simulink model "testemplanner_cs"  (R2020a)
settings: Solver=ode5  StartTime=0.0  StopTime=30  FixedStep=1/1000  RelTol=1e-3
PreLoadFcn:
  | mbxruntime.callbacks.PreLoadFcn(bdroot);
PostLoadFcn:
  | mbxruntime.callbacks.PostLoadFcn(bdroot);
InitFcn:
  | mbxruntime.callbacks.InitFcn(bdroot);
StartFcn:
  | mbxruntime.callbacks.StartFcn(bdroot);
StopFcn:
  | mbxruntime.callbacks.StopFcn(bdroot);
model workspace (MAT data in the model file):
  mbox_table : object (value not decoded)
  model_closed = 0
  sim_status = 0
values from neighbouring files (symbols this model uses):
  c_factor = 43.75    [emplanner_init.m]
  cf = -175016    [emplanner_init.m]
  cr = -130634    [emplanner_init.m]
  global_path_x = [-12.787 -11.7876177449 -10.7894946344 -9.79264775065 -8.79708287721 -7.80280164192 -6.80980414431 -5.81808992236 -4.82765830817 -3.83850855887 -2.85063990477 -1.86405156707 ... (3001 elements, 3001x1)]    [global_path.mat]
  global_path_y = [5.7602 5.7602 5.7602 5.7602 5.7602 5.7602 5.7602 5.7602 5.7602 5.7602 5.7602 5.7602 ... (3001 elements, 3001x1)]    [global_path.mat]
  KD_PID_distance = 0.0    (= 0)    [emplanner_init.m]
  KD_PID_speed = 0    [emplanner_init.m]
  KI_PID_distance = 0.0    (= 0)    [emplanner_init.m]
  KI_PID_speed = 0    [emplanner_init.m]
  KP_PID_distance = 0.5    [emplanner_init.m]
  KP_PID_speed = 1.8    [emplanner_init.m]
  la = 1.265    [emplanner_init.m]
  lb = 2.947-1.265    (= 1.682)    [emplanner_init.m]
  LQR_K1 = k(:,1)'    [emplanner_init.m]
  LQR_K2 = k(:,2)'    [emplanner_init.m]
  LQR_K3 = k(:,3)'    [emplanner_init.m]
  LQR_K4 = k(:,4)'    [emplanner_init.m]
  m = 2020    [emplanner_init.m]
  rack_displacement = [-39.14 , -37.2 , -35.29 , -33.43 , -31.6 , -29.81 , -28.06 , -26.34 , -24.66 ,      -23.01 , -21.38 , -19.79 , -18.23 , -16.69 , -15.18 , -13.7 , -12.23 , -10.8 , -9.38 , -7.98 ,     -6.61 , -5.25 , -3.91 , -2.59 , -1.29 , 0 , 1.27 , 2.54 , 3.78 , 5.02 , 6.24 , 7.46 , 8.66 ,      9.86 , 11.05 , 12.24 , 13.41 , 14.59 , 15.76 , 16.92 , 18.09 , 19.25 , 20.42 , 21.59 , 22.76 ,      23.93 , 25.11 , 26 ...(+26 chars)    [emplanner_init.m]
  right_wheel_ground = [-70 ,-67.2 , -64.4 , -61.6 , -58.8 , -56 , -53.2 , -50.4 , -47.6 , -44.8 , -42 ,      -39.2 , -36.4 , -33.6 , -30.8 , -28 , -25.2 , -22.4 , -19.6 , -16.8 , -14 , -11.2 , -8.4 , -5.6 ,      -2.8 , 0 , 2.8 , 5.6 , 8.4 , 11.2 , 14 , 16.8 , 19.6 , 22.4 , 25.2 , 28 , 30.8 , 33.6 , 36.4 ,      39.2 , 42 , 44.8 , 47.6 , 50.4 , 53.2 , 56 , 58.8 , 61.6 , 64.4 , 67.2 , 70 ]    [emplanner_init.m]
  vx_break_point = zeros(1,5000)    [emplanner_init.m]
undefined symbols (not defined in the file or in its folder): aubr, DiscIntNeverNeededParam, tablebr, vubr, warningInitialVelocity, x0
libraries: PreScanSimulinkLibrary x39, simulink x19, simulink_extras x11, Solver_SF x1
(part 5 of 16)

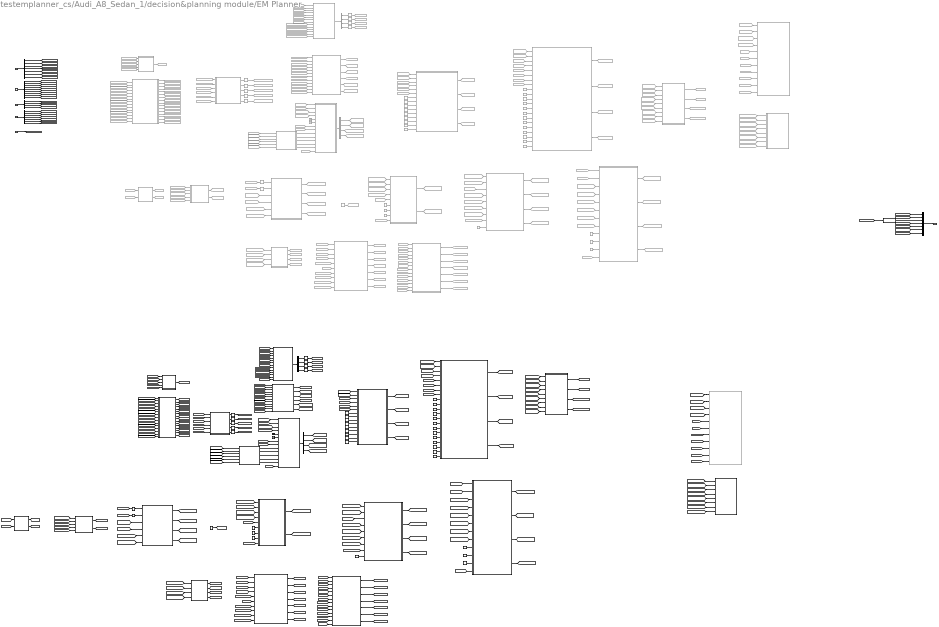
== system testemplanner_cs/Audi_A8_Sedan_1/decision&planning module/EM Planner ==
  referenceline info : Inport
  location info : Inport  Port=2
  perception info : Inport  Port=3
  pre_planning info : Inport  Port=4
  current time : Inport  Port=5
  Bus Creator : BusCreator  Inputs=7
  Bus Selector : BusSelector  OutputSignals=referenceline_x,referenceline_y,referenceline_heading,referenceline_kappa,origin_match_point_index,origin_x,origin_y
  Bus Selector1 : BusSelector  OutputSignals=host_x,host_y,host_heading_xy,host_vx,host_vy,host_yawrate,host_speed,host_ax,host_ay
  Bus Selector2 : BusSelector  OutputSignals=obs_x_set_gcs,obs_y_set_gcs,obs_velocity_set_gcs,obs_heading_set_gcs
  Bus Selector3 : BusSelector  OutputSignals=trajectory_x_gcs,trajectory_y_gcs,trajectory_heading_gcs,trajectory_kappa_gcs,trajectory_speed_gcs,trajectory_accel_gcs,trajectory_time_gcs
  Bus Selector4 : BusSelector  Commented=on  OutputSignals=s_set,l_set,dl_set,ddl_set
  Bus Selector5 : BusSelector  Commented=on  OutputSignals=s_set,l_set,s_dot_set,l_dot_set
  Bus Selector6 : BusSelector  OutputSignals=s_set,l_set,dl_set,ddl_set
  Bus Selector7 : BusSelector  OutputSignals=s_set,l_set,s_dot_set,l_dot_set
  Cartesian2Frenet : Subsystem  Commented=on
  Cartesian2Frenet1 : Subsystem  Commented=on
  Cartesian2Frenet2 : Subsystem
  Cartesian2Frenet3 : Subsystem
  Constant : Constant  Commented=on  Value=1e6
  Constant1 : Constant  Commented=on  Value=2000
  Constant10 : Constant  Commented=on  Value=0.1
  Constant11 : Constant  Commented=on  Value=0.02
  Constant12 : Constant  Commented=on  Value=2
  Constant13 : Constant  Commented=on  Value=25000
  Constant14 : Constant  Commented=on  Value=50
  Constant15 : Constant  Commented=on  Value=20
  Constant{7,16..19,23} (6 alike) : Constant  Commented=on  Value=15
  Constant2 : Constant  Commented=on  Value=2
  Constant20 : Constant  Commented=on  Value=3
  Constant21 : Constant  Commented=on  Value=3
  Constant22 : Constant  Commented=on  Value=1.63
  Constant24 : Constant  Commented=on  Value=4000
  Constant25 : Constant  Commented=on  Value=100
  Constant26 : Constant  Commented=on  Value=10000000
  Constant27 : Constant  Commented=on  Value=0.2*9.8
  Constant28 : Constant  Commented=on  Value=50
  Constant29 : Constant  Commented=on  Value=500
  Constant3 : Constant  Commented=on  Value=3
  Constant30 : Constant  Value=1e6
  Constant31 : Constant  Value=2000
  Constant32 : Constant  Value=0.1
  Constant33 : Constant  Value=0.02
  Constant34 : Constant  Value=2
  Constant35 : Constant  Value=25000
  Constant36 : Constant  Value=50
  Constant37 : Constant  Value=20
  Constant{38..41,46,57} (6 alike) : Constant  Value=15
  Constant4 : Constant  Commented=on  Value=10
  Constant42 : Constant  Value=2
  Constant43 : Constant  Value=3
  Constant44 : Constant  Value=3
  Constant45 : Constant  Value=1.63
  Constant47 : Constant  Value=4000
  Constant48 : Constant  Value=100
  Constant49 : Constant  Value=10000000
  Constant5 : Constant  Commented=on  Value=11
  Constant50 : Constant  Value=0.2*9.8
  Constant51 : Constant  Value=50
  Constant52 : Constant  Value=500
  Constant53 : Constant  Value=3
  Constant54 : Constant  Value=10
  Constant55 : Constant  Value=11
  Constant56 : Constant  Value=4
  Constant58 : Constant
  Constant59 : Constant  Value=10
  Constant6 : Constant  Commented=on  Value=4
  Constant8 : Constant  Commented=on
  Constant9 : Constant  Commented=on  Value=10
  Delay : Delay  Commented=on  DelayLength=1
  Delay1 : Delay  Commented=on  DelayLength=1
  Delay2 : Delay  DelayLength=1
  Delay3 : Delay  DelayLength=1
  Frenet2Cartesian : MATLAB Function  Commented=on  TreatAsAtomicUnit=on
  Frenet2Cartesian task : MATLAB Function  TreatAsAtomicUnit=on
  From : From  Commented=on  GotoTag=pre_trajectory_x_gcs
  From1 : From  Commented=on  GotoTag=pre_trajectory_y_gcs
  From10 : From  Commented=on  GotoTag=host_heading_xy
  From103 : From  Commented=on  GotoTag=trajectory_kappa_init
  From104 : From  Commented=on  GotoTag=plan_start_vx_gcs
  From105 : From  Commented=on  GotoTag=plan_start_vy_gcs
  From106 : From  Commented=on  GotoTag=plan_start_ax_gcs
  From107 : From  Commented=on  GotoTag=plan_start_ay_gcs
  From108 : From  Commented=on  GotoTag=plan_start_heading_gcs
  From109 : From  Commented=on  GotoTag=dynamic_obs_x_set
  From11 : From  Commented=on  GotoTag=host_vx_vcs
  From110 : From  Commented=on  GotoTag=stitch_x_gcs
  From111 : From  Commented=on  GotoTag=stitch_y_gcs
  From112 : From  Commented=on  GotoTag=stitch_heading_gcs
  From113 : From  Commented=on  GotoTag=stitch_kappa_gcs
  From114 : From  Commented=on  GotoTag=stitch_speed_gcs
  From115 : From  Commented=on  GotoTag=stitch_accel_gcs
  From116 : From  Commented=on  GotoTag=dynamic_obs_x_set
  From117 : From  Commented=on  GotoTag=dynamic_obs_y_set
  From118 : From  Commented=on  GotoTag=dynamic_obs_vx_set
  From119 : From  Commented=on  GotoTag=dynamic_obs_vy_set
  From12 : From  Commented=on  GotoTag=host_vy_vcs
  From120 : From  Commented=on  GotoTag=dynamic_obs_y_set
  From121 : From  Commented=on  GotoTag=s_dot2
  From122 : From  Commented=on  GotoTag=relative_time
  From{77,82,123,128} (4 alike) : From  Commented=on  GotoTag=trajectory_x_init
  From124 : From  Commented=on  GotoTag=dp_speed_s
  From125 : From  Commented=on  GotoTag=dp_speed_t
  From{78,83,91,127} (4 alike) : From  Commented=on  GotoTag=trajectory_y_init
  From{13,22,32,47,68} (5 alike) : From  Commented=on  GotoTag=referenceline_x
  From133 : From  Commented=on  GotoTag=dp_path_s_final
  From134 : From  Commented=on  GotoTag=dp_path_l_final
  From135 : From  Commented=on  GotoTag=l_min
  From136 : From  Commented=on  GotoTag=l_max
  From137 : From  Commented=on  GotoTag=plan_start_l
  From138 : From  Commented=on  GotoTag=plan_start_dl
  From139 : From  Commented=on  GotoTag=plan_start_s
  From{14,23,33,48,69} (5 alike) : From  Commented=on  GotoTag=referenceline_y
  From140 : From  Commented=on  GotoTag=static_obs_s_set
  From141 : From  Commented=on  GotoTag=static_obs_l_set
  From142 : From  Commented=on  GotoTag=qp_path_s_final
  From143 : From  Commented=on  GotoTag=qp_path_l_final
  From144 : From  Commented=on  GotoTag=path_index2s
  From145 : From  Commented=on  GotoTag=dynamic_obs_l_set
  From146 : From  Commented=on  GotoTag=dynamic_obs_s_dot_set
  From147 : From  Commented=on  GotoTag=dynamic_obs_l_dot_set
  From148 : From  Commented=on  GotoTag=obs_st_s_in_set
  From149 : From  Commented=on  GotoTag=obs_st_s_out_set
  From15 : From  Commented=on  GotoTag=host_ax_vcs
  From150 : From  Commented=on  GotoTag=relative_time
  From151 : From  Commented=on  GotoTag=s
  From152 : From  Commented=on  GotoTag=obs_st_t_in_set
  From153 : From  Commented=on  GotoTag=obs_st_t_out_set
  From154 : From  Commented=on  GotoTag=plan_start_s_dot
  From155 : From  Commented=on  GotoTag=path_index2s
  From156 : From  Commented=on  GotoTag=dp_speed_s
  From157 : From  Commented=on  GotoTag=dp_speed_t
  From158 : From  Commented=on  GotoTag=obs_st_s_in_set
  From159 : From  Commented=on  GotoTag=obs_st_s_out_set
  From16 : From  Commented=on  GotoTag=host_ay_vcs
  From160 : From  Commented=on  GotoTag=obs_st_t_in_set
  From161 : From  Commented=on  GotoTag=obs_st_t_out_set
  From162 : From  Commented=on  GotoTag=trajectory_kappa_init
  From163 : From  Commented=on  GotoTag=qp_s_init
  From164 : From  Commented=on  GotoTag=qp_s_dot_init
  From165 : From  Commented=on  GotoTag=obs_st_s_in_set
  From166 : From  Commented=on  GotoTag=obs_st_s_out_set
  From167 : From  Commented=on  GotoTag=obs_st_t_in_set
  From168 : From  Commented=on  GotoTag=obs_st_t_out_set
  From169 : From  Commented=on  GotoTag=dp_speed_s
  From17 : From  Commented=on  GotoTag=origin_x
  From170 : From  Commented=on  GotoTag=plan_start_s_dot
  From171 : From  Commented=on  GotoTag=plan_start_s_dot2
  From172 : From  Commented=on  GotoTag=dp_speed_t
  From173 : From  Commented=on  GotoTag=s_lb
  From174 : From  Commented=on  GotoTag=s_ub
  From175 : From  Commented=on  GotoTag=s_dot_lb
  From176 : From  Commented=on  GotoTag=s_dot_ub
  From177 : From  Commented=on  GotoTag=qp_s_init
  From178 : From  Commented=on  GotoTag=relative_time_init
  From179 : From  Commented=on  GotoTag=qp_s_dot2_init
  From18 : From  Commented=on  GotoTag=origin_y
  From180 : From  Commented=on  GotoTag=relative_time_init
  From186 : From  Commented=on  GotoTag=reference_speed
  From187 : From  Commented=on  GotoTag=reference_speed
  From19 : From  Commented=on  GotoTag=origin_match_point_index
  From2 : From  Commented=on  GotoTag=pre_trajectory_heading_gcs
  From20 : From  Commented=on  GotoTag=plan_start_x_gcs
  From21 : From  Commented=on  GotoTag=plan_start_y_gcs
  From24 : From  Commented=on  GotoTag=referenceline_heading
  From25 : From  Commented=on  GotoTag=referenceline_kappa
  From26 : From  Commented=on  GotoTag=plan_start_x_gcs
  From27 : From  Commented=on  GotoTag=plan_start_y_gcs
  From28 : From  Commented=on  GotoTag=plan_start_vx_gcs
  From29 : From  Commented=on  GotoTag=plan_start_vy_gcs
  From3 : From  Commented=on  GotoTag=pre_trajectory_kappa_gcs
  From30 : From  Commented=on  GotoTag=plan_start_ax_gcs
  From31 : From  Commented=on  GotoTag=plan_start_ay_gcs
  From34 : From  Commented=on  GotoTag=plan_start_match_point_index
  From35 : From  Commented=on  GotoTag=plan_start_proj_x
  From36 : From  Commented=on  GotoTag=plan_start_proj_y
  From37 : From  Commented=on  GotoTag=plan_start_proj_heading
  From38 : From  Commented=on  GotoTag=plan_start_proj_kappa
  From39 : From  Commented=on  GotoTag=index2s
  From4 : From  Commented=on  GotoTag=pre_trajectory_speed_gcs
  From40 : From  Commented=on  GotoTag=host_x
  From41 : From  Commented=on  GotoTag=host_y
  From42 : From  Commented=on  GotoTag=host_heading_xy
  From43 : From  Commented=on  GotoTag=obs_x_set_gcs
  From44 : From  Commented=on  GotoTag=obs_y_set_gcs
  From45 : From  Commented=on  GotoTag=obs_velocity_set_gcs
  From46 : From  Commented=on  GotoTag=obs_heading_set_gcs
  From49 : From  Commented=on  GotoTag=index2s
  From5 : From  Commented=on  GotoTag=pre_trajectory_accel_gcs
  From50 : From  Commented=on  GotoTag=referenceline_kappa
  From51 : From  Commented=on  GotoTag=referenceline_heading
  From52 : From  Commented=on  GotoTag=static_obs_s_set
  From53 : From  Commented=on  GotoTag=static_obs_l_set
  From54 : From  Commented=on  GotoTag=plan_start_s
  From55 : From  Commented=on  GotoTag=plan_start_l
  From56 : From  Commented=on  GotoTag=plan_start_dl
  From57 : From  Commented=on  GotoTag=plan_start_ddl
  From58 : From  Commented=on  GotoTag=dp_path_s_final
  From59 : From  Commented=on  GotoTag=dp_path_l_final
  From6 : From  Commented=on  GotoTag=pre_trajectory_time
  From60 : From  Commented=on  GotoTag=static_obs_s_set
  From61 : From  Commented=on  GotoTag=static_obs_l_set
  From62 : From  Commented=on  GotoTag=plan_start_l
  From63 : From  Commented=on  GotoTag=plan_start_dl
  From64 : From  Commented=on  GotoTag=dp_path_s_final
  From65 : From  Commented=on  GotoTag=dp_path_l_final
  From66 : From  Commented=on  GotoTag=dp_path_dl_final
  From67 : From  Commented=on  GotoTag=dp_path_ddl_final
  From7 : From  Commented=on  GotoTag=current_time
  From70 : From  Commented=on  GotoTag=referenceline_heading
  From71 : From  Commented=on  GotoTag=s
  From72 : From  Commented=on  GotoTag=s_dot
  From73 : From  Commented=on  GotoTag=path_index2s
  From74 : From  Commented=on  GotoTag=trajectory_x
  From75 : From  Commented=on  GotoTag=referenceline_kappa
  From76 : From  Commented=on  GotoTag=index2s
  From79 : From  Commented=on  GotoTag=trajectory_heading_init
  From8 : From  Commented=on  GotoTag=host_x
  From80 : From  Commented=on  GotoTag=trajectory_kappa_init
  From81 : From  Commented=on  GotoTag=dynamic_obs_s_set
  From84 : From  Commented=on  GotoTag=trajectory_y
  From85 : From  Commented=on  GotoTag=trajectory_heading
  From86 : From  Commented=on  GotoTag=trajectory_kappa
  From87 : From  Commented=on  GotoTag=trajectory_speed
  From88 : From  Commented=on  GotoTag=trajectory_accel
  From89 : From  Commented=on  GotoTag=trajectory_time
  From9 : From  Commented=on  GotoTag=host_y
  From90 : From  Commented=on  GotoTag=plan_start_ddl
  From92 : From  Commented=on  GotoTag=trajectory_heading_init
  From93 : From  Commented=on  GotoTag=plan_start_s
  From94 : From  Commented=on  GotoTag=stitch_time
  From95 : From  Commented=on  GotoTag=plan_start_time
  Goto100 : Goto  Commented=on  GotoTag=obs_st_t_in_set
  Goto101 : Goto  Commented=on  GotoTag=obs_st_t_out_set
  Goto102 : Goto  Commented=on  GotoTag=dp_speed_s
  Goto103 : Goto  Commented=on  GotoTag=dp_speed_t
  Goto104 : Goto  Commented=on  GotoTag=s_lb
  Goto105 : Goto  Commented=on  GotoTag=s_ub
  Goto106 : Goto  Commented=on  GotoTag=s_dot_lb
  Goto107 : Goto  Commented=on  GotoTag=s_dot_ub
  Goto108 : Goto  Commented=on  GotoTag=qp_s_init
  Goto109 : Goto  Commented=on  GotoTag=qp_s_dot_init
  Goto110 : Goto  Commented=on  GotoTag=qp_s_dot2_init
  Goto111 : Goto  Commented=on  GotoTag=relative_time_init
  Goto112 : Goto  Commented=on  GotoTag=reference_speed
  Goto25 : Goto  Commented=on  GotoTag=plan_start_x_gcs
  Goto26 : Goto  Commented=on  GotoTag=plan_start_y_gcs
  Goto27 : Goto  Commented=on  GotoTag=plan_start_heading_gcs
  Goto28 : Goto  Commented=on  GotoTag=plan_start_kappa_gcs
  Goto29 : Goto  Commented=on  GotoTag=plan_start_vx_gcs
  Goto30 : Goto  Commented=on  GotoTag=plan_start_vy_gcs
  Goto31 : Goto  Commented=on  GotoTag=plan_start_ax_gcs
  Goto32 : Goto  Commented=on  GotoTag=plan_start_ay_gcs
  Goto33 : Goto  Commented=on  GotoTag=plan_start_time
  Goto34 : Goto  Commented=on  GotoTag=stitch_x_gcs
  Goto35 : Goto  Commented=on  GotoTag=stitch_y_gcs
  Goto36 : Goto  Commented=on  GotoTag=stitch_heading_gcs
  Goto37 : Goto  Commented=on  GotoTag=stitch_kappa_gcs
  Goto38 : Goto  Commented=on  GotoTag=stitch_speed_gcs
  Goto39 : Goto  Commented=on  GotoTag=stitch_accel_gcs
  Goto40 : Goto  Commented=on  GotoTag=stitch_time
  Goto44 : Goto  Commented=on  GotoTag=index2s
  Goto45 : Goto  Commented=on  GotoTag=plan_start_match_point_index
  Goto46 : Goto  Commented=on  GotoTag=plan_start_proj_x
  Goto47 : Goto  Commented=on  GotoTag=plan_start_proj_y
  Goto48 : Goto  Commented=on  GotoTag=plan_start_proj_heading
  Goto49 : Goto  Commented=on  GotoTag=plan_start_proj_kappa
  Goto50 : Goto  Commented=on  GotoTag=plan_start_s
  Goto51 : Goto  Commented=on  GotoTag=plan_start_l
  Goto52 : Goto  Commented=on  GotoTag=plan_start_dl
  Goto53 : Goto  Commented=on  GotoTag=plan_start_ddl
  Goto54 : Goto  Commented=on  GotoTag=static_obs_s_set
  Goto55 : Goto  Commented=on  GotoTag=static_obs_l_set
  Goto56 : Goto  Commented=on  GotoTag=dynamic_obs_x_set
  Goto57 : Goto  Commented=on  GotoTag=dynamic_obs_y_set
  Goto58 : Goto  Commented=on  GotoTag=dp_path_s_final
  Goto59 : Goto  Commented=on  GotoTag=dp_path_l_final
  Goto60 : Goto  Commented=on  GotoTag=dp_path_dl_final
  Goto61 : Goto  Commented=on  GotoTag=dp_path_ddl_final
  Goto62 : Goto  Commented=on  GotoTag=trajectory_x_init
  Goto63 : Goto  Commented=on  GotoTag=trajectory_y_init
  Goto64 : Goto  Commented=on  GotoTag=trajectory_heading_init
  Goto65 : Goto  Commented=on  GotoTag=trajectory_kappa_init
  Goto66 : Goto  Commented=on  GotoTag=dynamic_obs_vx_set
  Goto67 : Goto  Commented=on  GotoTag=dynamic_obs_vy_set
  Goto68 : Goto  Commented=on  GotoTag=path_s_end
  Goto69 : Goto  Commented=on  GotoTag=path_index2s
  Goto70 : Goto  Commented=on  GotoTag=trajectory_x
  Goto71 : Goto  Commented=on  GotoTag=trajectory_y
  Goto72 : Goto  Commented=on  GotoTag=trajectory_heading
  Goto73 : Goto  Commented=on  GotoTag=trajectory_kappa
  Goto74 : Goto  Commented=on  GotoTag=trajectory_speed
  Goto75 : Goto  Commented=on  GotoTag=trajectory_accel
  Goto76 : Goto  Commented=on  GotoTag=plan_start_s_dot
  Goto77 : Goto  Commented=on  GotoTag=plan_start_s_dot2
  Goto78 : Goto  Commented=on  GotoTag=trajectory_time
  Goto79 : Goto  Commented=on  GotoTag=trajectory_x_final
  Goto80 : Goto  Commented=on  GotoTag=trajectory_y_final
  Goto81 : Goto  Commented=on  GotoTag=trajectory_heading_final
  Goto82 : Goto  Commented=on  GotoTag=trajectory_kappa_final
  Goto83 : Goto  Commented=on  GotoTag=trajectory_speed_final
  Goto84 : Goto  Commented=on  GotoTag=trajectory_accel_final
  Goto85 : Goto  Commented=on  GotoTag=trajectory_time_final
  Goto86 : Goto  Commented=on  GotoTag=dynamic_obs_s_set
  Goto87 : Goto  Commented=on  GotoTag=dynamic_obs_l_set
  Goto88 : Goto  Commented=on  GotoTag=dynamic_obs_s_dot_set
  Goto89 : Goto  Commented=on  GotoTag=qp_path_s_final
  Goto90 : Goto  Commented=on  GotoTag=qp_path_l_final
  Goto91 : Goto  Commented=on  GotoTag=qp_path_dl_final
  Goto92 : Goto  Commented=on  GotoTag=qp_path_ddl_final
  Goto93 : Goto  Commented=on  GotoTag=s
  Goto94 : Goto  Commented=on  GotoTag=s_dot
  Goto95 : Goto  Commented=on  GotoTag=s_dot2
  Goto96 : Goto  Commented=on  GotoTag=relative_time
  Goto97 : Goto  Commented=on  GotoTag=dynamic_obs_l_dot_set
  Goto98 : Goto  Commented=on  GotoTag=obs_st_s_in_set
  Goto99 : Goto  Commented=on  GotoTag=obs_st_s_out_set
  Ground : Ground  Commented=on
  Ground1 : Ground  Commented=on
  Ground2 : Ground
  Ground3 : Ground
  MATLAB Function : MATLAB Function  TreatAsAtomicUnit=on
  MATLAB Function1 : MATLAB Function  Commented=on  TreatAsAtomicUnit=on
  MATLAB Function2 : MATLAB Function  Commented=on  TreatAsAtomicUnit=on
  MATLAB Function3 : MATLAB Function  TreatAsAtomicUnit=on
  MATLAB Function4 : MATLAB Function  TreatAsAtomicUnit=on
  MATLAB Function5 : MATLAB Function  TreatAsAtomicUnit=on
  Selector{1..9} (9 alike) : Selector  Commented=on  InputPortWidth=128  IndexOptions=Index vector (dialog)  Indices=1  OutputSizes=1
  Selector{10..18} (9 alike) : Selector  InputPortWidth=128  IndexOptions=Index vector (dialog)  Indices=1  OutputSizes=1
  calc path length and map between point and s : MATLAB Function  Commented=on  TreatAsAtomicUnit=on
  calc path length and map between point and s1 : MATLAB Function  TreatAsAtomicUnit=on
  calc plan start info and stitch trajectory : MATLAB Function  Commented=on  TreatAsAtomicUnit=on
  calc plan start info and stitch trajectory1 : MATLAB Function  TreatAsAtomicUnit=on
  calc speed planning start condition : MATLAB Function  Commented=on  TreatAsAtomicUnit=on
  calc speed planning start condition1 : MATLAB Function  TreatAsAtomicUnit=on
  generate convex space : MATLAB Function  Commented=on  TreatAsAtomicUnit=on
  generate convex space1 : MATLAB Function  TreatAsAtomicUnit=on
  generate index to s : MATLAB Function  Commented=on  TreatAsAtomicUnit=on
  generate st graph : MATLAB Function  Commented=on  TreatAsAtomicUnit=on
  generate st graph1 : MATLAB Function  TreatAsAtomicUnit=on
  genrate index to s : MATLAB Function  TreatAsAtomicUnit=on
  increase st point count : MATLAB Function  Commented=on  TreatAsAtomicUnit=on
  increase st point count1 : MATLAB Function  TreatAsAtomicUnit=on
  obs : Subsystem  Commented=on
  obs1 : Subsystem
  path and speed merge : MATLAB Function  Commented=on  TreatAsAtomicUnit=on
  path and speed merge1 : MATLAB Function  TreatAsAtomicUnit=on
  path decision task : Subsystem  Commented=on
  path decision task1 : Subsystem
  path planning plot (SL) : MATLAB Function  Commented=on  TreatAsAtomicUnit=on
  path planning task : Subsystem  Commented=on
  path planning task1 : Subsystem
  plot : MATLAB Function  Commented=on  TreatAsAtomicUnit=on
  spee planning with quadratic programming (qp) : MATLAB Function  TreatAsAtomicUnit=on
  speed decision with dynamic planning(dp) : MATLAB Function  Commented=on  TreatAsAtomicUnit=on
  speed decision with dynamic planning(dp)1 : MATLAB Function  TreatAsAtomicUnit=on
  speed planning with quadratic programming (qp) : MATLAB Function  Commented=on  TreatAsAtomicUnit=on
  stitch trajectory : MATLAB Function  Commented=on  TreatAsAtomicUnit=on
  stitch trajectory1 : MATLAB Function  TreatAsAtomicUnit=on
  velocity planning plot (ST) : MATLAB Function  Commented=on  TreatAsAtomicUnit=on
  EM Planner result : Outport
  wires:
  location info/1 -> Bus Selector1/1
  Bus Selector/2 -> [referenceline_y]  "<referenceline_y>"
  Bus Selector/1 -> [referenceline_x]  "<referenceline_x>"
  Bus Selector3/5 -> [pre_trajectory_speed_gcs]  "<trajectory_speed_gcs>"
  Bus Selector2/3 -> [obs_velocity_set_gcs]  "<obs_velocity_set_gcs>"
  Bus Selector1/4 -> [host_vx_vcs]  "<host_vx>"
  Bus Selector1/9 -> [host_ay_vcs]  "<host_ay>"
  current time/1 -> [current_time]
  Bus Selector2/4 -> [obs_heading_set_gcs]  "<obs_heading_set_gcs>"
  Bus Selector/4 -> [referenceline_kappa]  "<referenceline_kappa>"
  Bus Selector/3 -> [referenceline_heading]  "<referenceline_heading>"
  Bus Selector1/6 -> [host_yawrate]  "<host_yawrate>"
  Bus Selector3/2 -> [pre_trajectory_y_gcs]  "<trajectory_y_gcs>"
  Bus Selector3/6 -> [pre_trajectory_accel_gcs]  "<trajectory_accel_gcs>"
  referenceline info/1 -> Bus Selector/1
  pre_planning info/1 -> Bus Selector3/1
  Bus Selector2/2 -> [obs_y_set_gcs]  "<obs_y_set_gcs>"
  Bus Selector3/3 -> [pre_trajectory_heading_gcs]  "<trajectory_heading_gcs>"
  Bus Selector3/1 -> [pre_trajectory_x_gcs]  "<trajectory_x_gcs>"
  perception info/1 -> Bus Selector2/1
  Bus Selector1/1 -> [host_x]  "<host_x>"
  Bus Selector3/7 -> [pre_trajectory_time]  "<trajectory_time_gcs>"
  Bus Selector3/4 -> [pre_trajectory_kappa_gcs]  "<trajectory_kappa_gcs>"
  Bus Selector1/2 -> [host_y]  "<host_y>"
  Bus Selector2/1 -> [obs_x_set_gcs]  "<obs_x_set_gcs>"
  Bus Selector1/7 -> [host_speed]  "<host_speed>"
  Bus Selector1/3 -> [host_heading_xy]  "<host_heading_xy>"
  Bus Selector1/5 -> [host_vy_vcs]  "<host_vy>"
  Bus Selector1/8 -> [host_ax_vcs]  "<host_ax>"
  From/1 -> calc plan start info and stitch trajectory/1(pre_trajectory_x)
  From1/1 -> calc plan start info and stitch trajectory/2(pre_trajectory_y)
  From2/1 -> calc plan start info and stitch trajectory/3(pre_trajectory_heading)
  From3/1 -> calc plan start info and stitch trajectory/4(pre_trajectory_kappa)
  From4/1 -> calc plan start info and stitch trajectory/5(pre_trajectory_velocity)
  From5/1 -> calc plan start info and stitch trajectory/6(pre_trajectory_accel)
  From6/1 -> calc plan start info and stitch trajectory/7(pre_trajectory_time)
  From7/1 -> calc plan start info and stitch trajectory/8(current_time)
  From8/1 -> calc plan start info and stitch trajectory/9(host_x)
  From9/1 -> calc plan start info and stitch trajectory/10(host_y)
  From10/1 -> calc plan start info and stitch trajectory/11(host_heading_xy)
  From11/1 -> calc plan start info and stitch trajectory/12(host_vx)
  From12/1 -> calc plan start info and stitch trajectory/13(host_vy)
  From15/1 -> calc plan start info and stitch trajectory/14(host_ax)
  From16/1 -> calc plan start info and stitch trajectory/15(host_ay)
  calc plan start info and stitch trajectory/16(stitch_time) -> Goto40/1
  calc plan start info and stitch trajectory/15(stitch_accel) -> Goto39/1
  calc plan start info and stitch trajectory/14(stitch_speed) -> Goto38/1
  calc plan start info and stitch trajectory/13(stitch_kappa) -> Goto37/1
  calc plan start info and stitch trajectory/12(stitch_heading) -> Goto36/1
  calc plan start info and stitch trajectory/11(stitch_y) -> Goto35/1
  calc plan start info and stitch trajectory/10(stitch_x) -> Goto34/1
  calc plan start info and stitch trajectory/9(plan_start_time) -> Goto33/1
  calc plan start info and stitch trajectory/8(plan_start_ay) -> Goto32/1
  calc plan start info and stitch trajectory/7(plan_start_ax) -> Goto31/1
  calc plan start info and stitch trajectory/6(plan_start_vy) -> Goto30/1
  calc plan start info and stitch trajectory/5(plan_start_vx) -> Goto29/1
  calc plan start info and stitch trajectory/4(plan_start_kappa) -> Goto28/1
  calc plan start info and stitch trajectory/3(plan_start_heading) -> Goto27/1
  calc plan start info and stitch trajectory/2(plan_start_y) -> Goto26/1
  calc plan start info and stitch trajectory/1(plan_start_x) -> Goto25/1
  Bus Selector/5 -> [origin_match_point_index]  "<origin_match_point_index>"
  Bus Selector/6 -> [origin_x]  "<origin_x>"
  Bus Selector/7 -> [origin_y]  "<origin_y>"
  From13/1 -> generate index to s/1(path_x)
  From14/1 -> generate index to s/2(path_y)
  From17/1 -> generate index to s/3(origin_x)
  From18/1 -> generate index to s/4(origin_y)
  From19/1 -> generate index to s/5(origin_match_point_index)
  generate index to s/1(index2s) -> Goto44/1
  Selector1/1 -> Goto45/1
  Selector2/1 -> Goto46/1
  Selector3/1 -> Goto47/1
  Selector4/1 -> Goto48/1
  Selector5/1 -> Goto49/1
  From26/1 -> Cartesian2Frenet/1(x_set)
  From27/1 -> Cartesian2Frenet/2(y_set)
  From28/1 -> Cartesian2Frenet/3(vx_set)
  From29/1 -> Cartesian2Frenet/4(vy_set)
  From30/1 -> Cartesian2Frenet/5(ax_set)
  From31/1 -> Cartesian2Frenet/6(ay_set)
  From32/1 -> Cartesian2Frenet/7(frenet_path_x)
  From33/1 -> Cartesian2Frenet/8(frenet_path_y)
  From34/1 -> Cartesian2Frenet/9(proj_match_point_index_set)
  From35/1 -> Cartesian2Frenet/10(proj_x_set)
  From36/1 -> Cartesian2Frenet/11(proj_y_set)
  From37/1 -> Cartesian2Frenet/12(proj_heading_set)
  From38/1 -> Cartesian2Frenet/13(proj_kappa_set)
  From39/1 -> Cartesian2Frenet/14(index2s)
  Bus Selector4/2 -> Selector7/1  "<l_set>"
  Selector9/1 -> Goto53/1
  Selector6/1 -> Goto50/1
  Selector8/1 -> Goto52/1
  Selector7/1 -> Goto51/1
  Bus Selector4/1 -> Selector6/1  "<s_set>"
  Bus Selector4/3 -> Selector8/1  "<dl_set>"
  Bus Selector4/4 -> Selector9/1  "<ddl_set>"
  Cartesian2Frenet/1(Cartesian2FrenetOut) -> Bus Selector4/1
  From49/1 -> obs/12(index2s)
  From50/1 -> obs/11(referenceline_kappa)
  From51/1 -> obs/10(referenceline_heading)
  From48/1 -> obs/9(referenceline_y)
  From47/1 -> obs/8(referenceline_x)
  From46/1 -> obs/7(obs_heading_set_gcs)
  From45/1 -> obs/6(obs_velocity_set_gcs)
  From44/1 -> obs/5(obs_y_set_gcs)
  From43/1 -> obs/4(obs_x_set_gcs)
  From42/1 -> obs/3(host_heading_xy)
  From41/1 -> obs/2(host_y)
  From40/1 -> obs/1(host_x)
  obs/1(static_obs_s_set) -> Goto54/1
  obs/2(static_obs_l_set) -> Goto55/1
  From76/1 -> Frenet2Cartesian/9(index2s)
  From64/1 -> Frenet2Cartesian/1(s_set)
  Frenet2Cartesian/1(x_set) -> Goto62/1
  Frenet2Cartesian/4(kappa_set) -> Goto65/1
  Frenet2Cartesian/3(heading_set) -> Goto64/1
  From75/1 -> Frenet2Cartesian/8(frenet_path_kappa)
  From70/1 -> Frenet2Cartesian/7(frenet_path_heading)
  Frenet2Cartesian/2(y_set) -> Goto63/1
  From69/1 -> Frenet2Cartesian/6(frenet_path_y)
  From68/1 -> Frenet2Cartesian/5(frenet_path_x)
  From65/1 -> Frenet2Cartesian/2(l_set)
  From66/1 -> Frenet2Cartesian/3(dl_set)
  From67/1 -> Frenet2Cartesian/4(ddl_set)
  [trajectory_speed_final] -> Bus Creator/5  "trajectory_speed_gcs"
  [trajectory_y_final] -> Bus Creator/2  "trajectory_y_gcs"
  [trajectory_time_final] -> Bus Creator/7  "trajectory_time_gcs"
  [trajectory_accel_final] -> Bus Creator/6  "trajectory_accel_gcs"
  [trajectory_kappa_final] -> Bus Creator/4  "trajectory_kappa_gcs"
  [trajectory_x_final] -> Bus Creator/1  "trajectory_x_gcs"
  From20/1 -> MATLAB Function1/1(x_set)
  From21/1 -> MATLAB Function1/2(y_set)
  From22/1 -> MATLAB Function1/3(frenet_path_x)
  From23/1 -> MATLAB Function1/4(frenet_path_y)
  From24/1 -> MATLAB Function1/5(frenet_path_heading)
  From25/1 -> MATLAB Function1/6(frenet_path_kappa)
  MATLAB Function1/5(proj_kappa_set) -> Selector5/1
  MATLAB Function1/4(proj_heading_set) -> Selector4/1
  MATLAB Function1/3(proj_y_set) -> Selector3/1
  MATLAB Function1/2(proj_x_set) -> Selector2/1
  MATLAB Function1/1(match_point_index_set) -> Selector1/1
  From135/1 -> path planning plot (SL)/5(l_min)
  From143/1 -> path planning plot (SL)/4(qp_l)
  From141/1 -> path planning plot (SL)/8(obs_l_set)
  From136/1 -> path planning plot (SL)/6(l_max)
  From142/1 -> path planning plot (SL)/3(qp_s)
  From139/1 -> path planning plot (SL)/9(start_s)
  From138/1 -> path planning plot (SL)/11(start_dl)
  From134/1 -> path planning plot (SL)/2(dp_l)
  From137/1 -> path planning plot (SL)/10(start_l)
  From133/1 -> path planning plot (SL)/1(dp_s)
  From140/1 -> path planning plot (SL)/7(obs_s_set)
  path decision task/1(dp_path_s_final) -> Goto58/1
  path decision task/2(dp_path_l_final) -> Goto59/1
  path decision task/3(dp_path_dl_final) -> Goto60/1
  path decision task/4(dp_path_ddl_final) -> Goto61/1
  From52/1 -> path decision task/1(static_obs_s_set)
  From53/1 -> path decision task/2(static_obs_l_set)
  From54/1 -> path decision task/3(plan_start_s)
  From55/1 -> path decision task/4(plan_start_l)
  From56/1 -> path decision task/5(plan_start_dl)
  From57/1 -> path decision task/6(plan_start_ddl)
  Constant/1 -> path decision task/7(dp_cost_collision)
  Constant1/1 -> path decision task/8(dp_cost_dl)
  Constant2/1 -> path decision task/9(dp_cost_ddl)
  Constant3/1 -> path decision task/10(dp_cost_dddl)
  Constant4/1 -> path decision task/11(dp_cost_ref)
  Constant5/1 -> path decision task/12(dp_row)
  Constant6/1 -> path decision task/13(dp_col)
  Constant7/1 -> path decision task/14(dp_sample_s)
  Constant8/1 -> path decision task/15(dp_sample_l)
  From59/1 -> path planning task/2(dp_path_l_final1)
  From58/1 -> path planning task/1(dp_path_s_final)
  From60/1 -> path planning task/3(static_obs_s_set)
  From61/1 -> path planning task/4(static_obs_l_set)
  From93/1 -> path planning task/5(plan_start_s)
  From62/1 -> path planning task/6(plan_start_l)
  From63/1 -> path planning task/7(plan_start_dl)
  From90/1 -> path planning task/8(plan_start_ddl)
  Constant11/1 -> path planning task/21(delta_ddl_max)
  Constant10/1 -> path planning task/20(delta_dl_max)
  Constant22/1 -> path planning task/19(host_w)
  Constant20/1 -> path planning task/17(host_d1)
  Constant21/1 -> path planning task/18(host_d2)
  Constant19/1 -> path planning task/16(qp_cost_end_ddl)
  Constant18/1 -> path planning task/15(qp_cost_end_dl)
  Constant17/1 -> path planning task/14(qp_cost_endl)
  Constant16/1 -> path planning task/13(qp_cost_centre)
  Constant15/1 -> path planning task/12(qp_cost_dddl)
  Constant14/1 -> path planning task/11(qp_cost_ddl)
  Constant13/1 -> path planning task/10(qp_cost_dl)
  Constant12/1 -> path planning task/9(qp_cost_l)
  path planning task/1(qp_path_s_final) -> Goto89/1
  path planning task/2(qp_path_l_final) -> Goto90/1
  path planning task/4(qp_path_ddl_final) -> Goto92/1
  path planning task/3(qp_path_dl_final) -> Goto91/1
  MATLAB Function/1(y) -> Bus Creator/3  "trajectory_heading_gcs"
  [trajectory_heading_final] -> MATLAB Function/1(trajectory_heading_final)  "trajectory_heading_gcs"
  obs/3(dynamic_obs_x_set) -> Goto56/1
  obs/4(dynamic_obs_y_set) -> Goto57/1
  obs/5(dynamic_obs_vx_set) -> Goto66/1
  obs/6(dynamic_obs_vy_set) -> Goto67/1
  From77/1 -> calc path length and map between point and s/1(trajectory_x)
  From78/1 -> calc path length and map between point and s/2(trajectory_y)
  calc path length and map between point and s/2(path_index2s) -> Goto69/1
  calc path length and map between point and s/1(path_s_end) -> Goto68/1
  Bus Selector5/1 -> Goto86/1  "<s_set>"
  MATLAB Function2/3(proj_y_set) -> Cartesian2Frenet1/11(proj_y_set)
  From144/1 -> Cartesian2Frenet1/14(index2s)
  MATLAB Function2/5(proj_kappa_set) -> Cartesian2Frenet1/13(proj_kappa_set)
  From127/1 -> Cartesian2Frenet1/8(frenet_path_y)
  From123/1 -> Cartesian2Frenet1/7(frenet_path_x)
  From119/1 -> Cartesian2Frenet1/4(vy_set)
  Bus Selector5/2 -> Goto87/1  "<l_set>"
  MATLAB Function2/4(proj_heading_set) -> Cartesian2Frenet1/12(proj_heading_set)
  Cartesian2Frenet1/1(Cartesian2FrenetOut) -> Bus Selector5/1
  Ground1/1 -> Cartesian2Frenet1/6(ay_set)
  MATLAB Function2/2(proj_x_set) -> Cartesian2Frenet1/10(proj_x_set)
  Ground/1 -> Cartesian2Frenet1/5(ax_set)
  MATLAB Function2/1(match_point_index_set) -> Cartesian2Frenet1/9(proj_match_point_index_set)
  From116/1 -> Cartesian2Frenet1/1(x_set)
  From117/1 -> Cartesian2Frenet1/2(y_set)
  Bus Selector5/3 -> Goto88/1  "<s_dot_set>"
  From118/1 -> Cartesian2Frenet1/3(vx_set)
  Bus Selector5/4 -> Goto97/1  "<l_dot_set>"
  From120/1 -> MATLAB Function2/2(y_set)
  From92/1 -> MATLAB Function2/5(frenet_path_heading)
  From91/1 -> MATLAB Function2/4(frenet_path_y)
  From109/1 -> MATLAB Function2/1(x_set)
  From103/1 -> MATLAB Function2/6(frenet_path_kappa)
  From128/1 -> MATLAB Function2/3(frenet_path_x)
  calc speed planning start condition/2(plan_start_s_dot2) -> Goto77/1
  From107/1 -> calc speed planning start condition/4(plan_start_ay)
  calc speed planning start condition/1(plan_start_s_dot) -> Goto76/1
  From104/1 -> calc speed planning start condition/1(plan_start_vx)
  From105/1 -> calc speed planning start condition/2(plan_start_vy)
  From108/1 -> calc speed planning start condition/5(plan_start_heading)
  From106/1 -> calc speed planning start condition/3(plan_start_ax)
  From145/1 -> generate st graph/4(dynamic_obs_l_set)
  generate st graph/2(obs_st_s_out_set) -> Goto99/1
  From147/1 -> generate st graph/6(dynamic_obs_l_dot_set)
  From146/1 -> generate st graph/5(dynamic_obs_s_dot_set)
  From81/1 -> generate st graph/3(dynamic_obs_s_set)
  From150/1 -> Delay1/1
  Delay1/1 -> generate st graph/2(pre_trajectory_t)
  generate st graph/3(obs_st_t_in_set) -> Goto100/1
  From151/1 -> Delay/1
  generate st graph/1(obs_st_s_in_set) -> Goto98/1
  generate st graph/4(obs_st_t_out_set) -> Goto101/1
  Delay/1 -> generate st graph/1(pre_trajectory_s)
  speed decision with dynamic planning(dp)/2(dp_speed_t) -> Goto103/1
  From152/1 -> speed decision with dynamic planning(dp)/3(obs_st_t_in_set)
  From153/1 -> speed decision with dynamic planning(dp)/4(obs_st_t_out_set)
  Constant26/1 -> speed decision with dynamic planning(dp)/8(w_cost_obs)
  From148/1 -> speed decision with dynamic planning(dp)/1(obs_st_s_in_set)
  Constant23/1 -> Goto112/1
  speed decision with dynamic planning(dp)/1(dp_speed_s) -> Goto102/1
  Constant24/1 -> speed decision with dynamic planning(dp)/6(w_cost_ref_speed)
  From186/1 -> speed decision with dynamic planning(dp)/5(reference_speed_unlimit)
  Constant25/1 -> speed decision with dynamic planning(dp)/7(w_cost_accel)
  From154/1 -> speed decision with dynamic planning(dp)/9(plan_start_s_dot)
  From149/1 -> speed decision with dynamic planning(dp)/2(obs_st_s_out_set)
  From155/1 -> generate convex space/3(path_index2s)
  From159/1 -> generate convex space/5(obs_st_s_out_set)
  generate convex space/4(s_dot_ub) -> Goto107/1
  generate convex space/2(s_ub) -> Goto105/1
  From158/1 -> generate convex space/4(obs_st_s_in_set)
  From162/1 -> generate convex space/8(trajectory_kappa_init)
  From161/1 -> generate convex space/7(obs_st_t_out_set)
  From157/1 -> generate convex space/2(dp_speed_t)
  generate convex space/1(s_lb) -> Goto104/1
  From156/1 -> generate convex space/1(dp_speed_s)
  generate convex space/3(s_dot_lb) -> Goto106/1
  From160/1 -> generate convex space/6(obs_st_t_in_set)
  Constant27/1 -> generate convex space/9(max_lateral_accel)
  From169/1 -> speed planning with quadratic programming (qp)/3(dp_speed_s)
  Constant28/1 -> speed planning with quadratic programming (qp)/10(w_cost_v_ref)
  From187/1 -> speed planning with quadratic programming (qp)/12(speed_reference)
  Constant29/1 -> speed planning with quadratic programming (qp)/11(w_cost_jerk)
  From170/1 -> speed planning with quadratic programming (qp)/1(plan_start_s_dot)
  From171/1 -> speed planning with quadratic programming (qp)/2(plan_start_s_dot2)
  speed planning with quadratic programming (qp)/4(relative_time_init) -> Goto111/1
  speed planning with quadratic programming (qp)/3(qp_s_dot2_init) -> Goto110/1
  From175/1 -> speed planning with quadratic programming (qp)/7(s_dot_lb)
  From174/1 -> speed planning with quadratic programming (qp)/6(s_ub)
  From176/1 -> speed planning with quadratic programming (qp)/8(s_dot_ub)
  speed planning with quadratic programming (qp)/1(qp_s_init) -> Goto108/1
  speed planning with quadratic programming (qp)/2(qp_s_dot_init) -> Goto109/1
  From173/1 -> speed planning with quadratic programming (qp)/5(s_lb)
  Constant9/1 -> speed planning with quadratic programming (qp)/9(w_cost_s_dot2)
  From172/1 -> speed planning with quadratic programming (qp)/4(dp_speed_t)
  From95/1 -> path and speed merge/5(current_time)
  From113/1 -> stitch trajectory/11(stitch_kappa)
  From83/1 -> path and speed merge/8(trajectory_y_init)
  From89/1 -> stitch trajectory/7(trajectory_time)
  stitch trajectory/4(trajectory_kappa_final) -> Goto82/1
  From112/1 -> stitch trajectory/10(stitch_heading)
  path and speed merge/7(trajectory_time) -> Goto78/1
  stitch trajectory/1(trajectory_x_final) -> Goto79/1
  From86/1 -> stitch trajectory/4(trajectory_kappa)
  path and speed merge/1(trajectory_x) -> Goto70/1
  From73/1 -> path and speed merge/6(path_s)
  path and speed merge/3(trajectory_heading) -> Goto72/1
  stitch trajectory/3(trajectory_heading_final) -> Goto81/1
  stitch trajectory/2(trajectory_y_final) -> Goto80/1
  increase st point count/4(relative_time) -> Goto96/1
  From110/1 -> stitch trajectory/8(stitch_x)
  path and speed merge/5(trajectory_speed) -> Goto74/1
  increase st point count/3(s_dot2) -> Goto95/1
  stitch trajectory/6(trajectory_accel_final) -> Goto84/1
  From164/1 -> increase st point count/2(s_dot_init)
  From82/1 -> path and speed merge/7(trajectory_x_init)
  From111/1 -> stitch trajectory/9(stitch_y)
  From115/1 -> stitch trajectory/13(stitch_accel)
  From88/1 -> stitch trajectory/6(trajectory_accel)
  path and speed merge/2(trajectory_y) -> Goto71/1
  path and speed merge/6(trajectory_accel) -> Goto75/1
  From84/1 -> stitch trajectory/2(trajectory_y)
  From94/1 -> stitch trajectory/14(stitch_time)
  stitch trajectory/7(trajectory_time_final) -> Goto85/1
  stitch trajectory/5(trajectory_speed_final) -> Goto83/1
  From80/1 -> path and speed merge/10(trajectory_kappa_init)
  From74/1 -> stitch trajectory/1(trajectory_x)
  From71/1 -> path and speed merge/1(s)
  increase st point count/2(s_dot) -> Goto94/1
  From85/1 -> stitch trajectory/3(trajectory_heading)
  From180/1 -> increase st point count/4(relative_time_init)
  From114/1 -> stitch trajectory/12(stitch_speed)
  From87/1 -> stitch trajectory/5(trajectory_speed)
  From72/1 -> path and speed merge/2(s_dot)
  From79/1 -> path and speed merge/9(trajectory_heading_init)
  From163/1 -> increase st point count/1(s_init)
  path and speed merge/4(trajectory_kappa) -> Goto73/1
  From179/1 -> increase st point count/3(s_dot2_init)
  From121/1 -> path and speed merge/3(s_dot2)
  increase st point count/1(s) -> Goto93/1
  From122/1 -> path and speed merge/4(relative_time)
  From124/1 -> velocity planning plot (ST)/1(dp_speed_s)
  From167/1 -> velocity planning plot (ST)/7(obs_t_in_set)
  From125/1 -> velocity planning plot (ST)/2(dp_speed_t)
  From165/1 -> velocity planning plot (ST)/5(obs_s_in_set)
  From166/1 -> velocity planning plot (ST)/6(obs_s_out_set)
  From168/1 -> velocity planning plot (ST)/8(obs_t_out_set)
  From178/1 -> velocity planning plot (ST)/4(qp_speed_t)
  From177/1 -> velocity planning plot (ST)/3(qp_speed_s)
  Bus Creator/1 -> EM Planner result/1
  [host_vx_vcs] -> calc plan start info and stitch trajectory1/12(host_vx)
  [host_vy_vcs] -> calc plan start info and stitch trajectory1/13(host_vy)
  [host_ax_vcs] -> calc plan start info and stitch trajectory1/14(host_ax)
  Constant57/1 -> path decision task1/14(dp_sample_s)
  Selector14/1 -> [plan_start_proj_kappa]
  [referenceline_kappa] -> Frenet2Cartesian task/8(frenet_path_kappa)
  calc path length and map between point and s1/2(path_index2s) -> [path_index2s]
  Constant34/1 -> path planning task1/9(qp_cost_l)
  Constant36/1 -> path planning task1/11(qp_cost_ddl)
  calc plan start info and stitch trajectory1/4(plan_start_kappa) -> [plan_start_kappa_gcs]
  [plan_start_dl] -> path decision task1/5(plan_start_dl)
  [static_obs_s_set] -> path decision task1/1(static_obs_s_set)
  Constant38/1 -> path planning task1/13(qp_cost_centre)
  [plan_start_ddl] -> path planning task1/8(plan_start_ddl)
  path decision task1/2(dp_path_l_final) -> [dp_path_l_final]
  [dp_path_s_final] -> path planning task1/1(dp_path_s_final)
  [plan_start_ddl] -> path decision task1/6(plan_start_ddl)
  [dp_path_s_final] -> plot/1(dp_s)
  path and speed merge1/7(trajectory_time) -> [trajectory_time]
  Constant45/1 -> path planning task1/19(host_w)
  Constant37/1 -> path planning task1/12(qp_cost_dddl)
  MATLAB Function4/3(proj_y_set) -> Selector12/1
  [obs_heading_set_gcs] -> obs1/7(obs_heading_set_gcs)
  [static_obs_s_set] -> plot/7(obs_s_set)
  Frenet2Cartesian task/1(x_set) -> [trajectory_x_init]
  [plan_start_l] -> plot/10(start_l)
  Frenet2Cartesian task/4(kappa_set) -> [trajectory_kappa_init]
  [dp_path_l_final] -> plot/2(dp_l)
  [plan_start_s] -> plot/9(start_s)
  [plan_start_dl] -> plot/11(start_dl)
  path decision task1/1(dp_path_s_final) -> [dp_path_s_final]
  [obs_x_set_gcs] -> obs1/4(obs_x_set_gcs)
  [referenceline_x] -> Frenet2Cartesian task/5(frenet_path_x)
  [trajectory_y_init] -> calc path length and map between point and s1/2(trajectory_y)
  [trajectory_x_init] -> calc path length and map between point and s1/1(trajectory_x)
  [obs_velocity_set_gcs] -> obs1/6(obs_velocity_set_gcs)
  [stitch_kappa_gcs] -> stitch trajectory1/11(stitch_kappa)
  obs1/1(static_obs_s_set) -> [static_obs_s_set]
  [trajectory_y_init] -> path and speed merge1/8(trajectory_y_init)
  [path_index2s] -> path and speed merge1/6(path_s)
  [trajectory_time] -> stitch trajectory1/7(trajectory_time)
  [trajectory_speed] -> stitch trajectory1/5(trajectory_speed)
  stitch trajectory1/4(trajectory_kappa_final) -> [trajectory_kappa_final]
  stitch trajectory1/1(trajectory_x_final) -> [trajectory_x_final]
  Selector16/1 -> [plan_start_l]
  calc speed planning start condition1/2(plan_start_s_dot2) -> [plan_start_s_dot2]
  path and speed merge1/1(trajectory_x) -> [trajectory_x]
  stitch trajectory1/3(trajectory_heading_final) -> [trajectory_heading_final]
  stitch trajectory1/2(trajectory_y_final) -> [trajectory_y_final]
  [stitch_y_gcs] -> stitch trajectory1/9(stitch_y)
  calc path length and map between point and s1/1(path_s_end) -> [path_s_end]
  [referenceline_y] -> obs1/9(referenceline_y)
  [referenceline_kappa] -> obs1/11(referenceline_kappa)
  [referenceline_y] -> Cartesian2Frenet2/8(frenet_path_y)
  [plan_start_match_point_index] -> Cartesian2Frenet2/9(proj_match_point_index_set)
  Bus Selector6/2 -> Selector16/1  "<l_set>"
  [static_obs_l_set] -> path decision task1/2(static_obs_l_set)
  Cartesian2Frenet2/1(Cartesian2FrenetOut) -> Bus Selector6/1
  Bus Selector6/4 -> Selector18/1  "<ddl_set>"
  [referenceline_x] -> obs1/8(referenceline_x)
  [obs_y_set_gcs] -> obs1/5(obs_y_set_gcs)
  [dp_path_l_final] -> path planning task1/2(dp_path_l_final)
  calc plan start info and stitch trajectory1/16(stitch_time) -> [stitch_time]
  Constant58/1 -> path decision task1/15(dp_sample_l)
  [plan_start_proj_kappa] -> Cartesian2Frenet2/13(proj_kappa_set)
  [host_heading_xy] -> obs1/3(host_heading_xy)
  [plan_start_time] -> path and speed merge1/5(current_time)
  Selector15/1 -> [plan_start_s]
  Selector10/1 -> [plan_start_match_point_index]
  [referenceline_kappa] -> MATLAB Function4/6(frenet_path_kappa)
  [plan_start_x_gcs] -> Cartesian2Frenet2/1(x_set)
  calc plan start info and stitch trajectory1/13(stitch_kappa) -> [stitch_kappa_gcs]
  Selector11/1 -> [plan_start_proj_x]
  [referenceline_x] -> MATLAB Function4/3(frenet_path_x)
  [plan_start_x_gcs] -> MATLAB Function4/1(x_set)
  [referenceline_y] -> MATLAB Function4/4(frenet_path_y)
  MATLAB Function4/4(proj_heading_set) -> Selector13/1
  Selector13/1 -> [plan_start_proj_heading]
  [plan_start_y_gcs] -> Cartesian2Frenet2/2(y_set)
  [referenceline_x] -> Cartesian2Frenet2/7(frenet_path_x)
  Selector12/1 -> [plan_start_proj_y]
  calc plan start info and stitch trajectory1/1(plan_start_x) -> [plan_start_x_gcs]
  [pre_trajectory_speed_gcs] -> calc plan start info and stitch trajectory1/5(pre_trajectory_velocity)
  [origin_match_point_index] -> genrate index to s/5(origin_match_point_index)
  calc plan start info and stitch trajectory1/12(stitch_heading) -> [stitch_heading_gcs]
  [origin_x] -> genrate index to s/3(origin_x)
  calc plan start info and stitch trajectory1/9(plan_start_time) -> [plan_start_time]
  [pre_trajectory_heading_gcs] -> calc plan start info and stitch trajectory1/3(pre_trajectory_heading)
  calc plan start info and stitch trajectory1/6(plan_start_vy) -> [plan_start_vy_gcs]
  [origin_y] -> genrate index to s/4(origin_y)
  [host_y] -> calc plan start info and stitch trajectory1/10(host_y)
  [current_time] -> calc plan start info and stitch trajectory1/8(current_time)
  Constant39/1 -> path planning task1/14(qp_cost_endl)
  [pre_trajectory_x_gcs] -> calc plan start info and stitch trajectory1/1(pre_trajectory_x)
  speed decision with dynamic planning(dp)1/2(dp_speed_t) -> [dp_speed_t]
  [obs_st_t_in_set] -> speed decision with dynamic planning(dp)1/3(obs_st_t_in_set)
  obs1/5(dynamic_obs_vx_set) -> [dynamic_obs_vx_set]
  [dp_speed_s] -> spee planning with quadratic programming (qp)/3(dp_speed_s)
  [referenceline_heading] -> Frenet2Cartesian task/7(frenet_path_heading)
  increase st point count1/4(relative_time) -> [relative_time]
  obs1/6(dynamic_obs_vy_set) -> [dynamic_obs_vy_set]
  [stitch_x_gcs] -> stitch trajectory1/8(stitch_x)
  Constant51/1 -> spee planning with quadratic programming (qp)/10(w_cost_v_ref)
  Constant40/1 -> path planning task1/15(qp_cost_end_dl)
  path and speed merge1/5(trajectory_speed) -> [trajectory_speed]
  increase st point count1/1(s) -> [s]
  [reference_speed] -> spee planning with quadratic programming (qp)/12(speed_reference)
  MATLAB Function4/5(proj_kappa_set) -> Selector14/1
  [static_obs_l_set] -> plot/8(obs_l_set)
  Constant53/1 -> path decision task1/10(dp_cost_dddl)
  stitch trajectory1/6(trajectory_accel_final) -> [trajectory_accel_final]
  Constant52/1 -> spee planning with quadratic programming (qp)/11(w_cost_jerk)
  Constant35/1 -> path planning task1/10(qp_cost_dl)
  [obs_st_s_out_set] -> generate convex space1/5(obs_st_s_out_set)
  [qp_path_l_final] -> plot/4(qp_l)
  [qp_s_dot_init] -> increase st point count1/2(s_dot_init)
  [plan_start_s_dot] -> spee planning with quadratic programming (qp)/1(plan_start_s_dot)
  [plan_start_proj_heading] -> Cartesian2Frenet2/12(proj_heading_set)
  Constant48/1 -> speed decision with dynamic planning(dp)1/7(w_cost_accel)
  Bus Selector6/1 -> Selector15/1  "<s_set>"
  Constant30/1 -> path decision task1/7(dp_cost_collision)
  [plan_start_s_dot2] -> spee planning with quadratic programming (qp)/2(plan_start_s_dot2)
  [plan_start_vx_gcs] -> Cartesian2Frenet2/3(vx_set)
  MATLAB Function3/3(proj_y_set) -> Cartesian2Frenet3/11(proj_y_set)
  [referenceline_heading] -> obs1/10(referenceline_heading)
  [plan_start_proj_x] -> Cartesian2Frenet2/10(proj_x_set)
  generate convex space1/3(s_dot_lb) -> [s_dot_lb]
  [plan_start_ay_gcs] -> calc speed planning start condition1/4(plan_start_ay)
  spee planning with quadratic programming (qp)/4(relative_time_init) -> [relative_time_init]
  spee planning with quadratic programming (qp)/3(qp_s_dot2_init) -> [qp_s_dot2_init]
  Constant44/1 -> path planning task1/18(host_d2)
  calc plan start info and stitch trajectory1/7(plan_start_ax) -> [plan_start_ax_gcs]
  spee planning with quadratic programming (qp)/1(qp_s_init) -> [qp_s_init]
  path planning task1/1(qp_path_s_final) -> [qp_path_s_final]
  [plan_start_s] -> path decision task1/3(plan_start_s)
  [stitch_accel_gcs] -> stitch trajectory1/13(stitch_accel)
  [s_dot_ub] -> spee planning with quadratic programming (qp)/8(s_dot_ub)
  [s_dot_lb] -> spee planning with quadratic programming (qp)/7(s_dot_lb)
  [trajectory_accel] -> stitch trajectory1/6(trajectory_accel)
  [dynamic_obs_s_dot_set] -> generate st graph1/5(dynamic_obs_s_dot_set)
  [referenceline_y] -> genrate index to s/2(path_y)
  [referenceline_y] -> Frenet2Cartesian task/6(frenet_path_y)
  path and speed merge1/2(trajectory_y) -> [trajectory_y]
  [host_y] -> obs1/2(host_y)
  Selector18/1 -> [plan_start_ddl]
  [dp_speed_t] -> spee planning with quadratic programming (qp)/4(dp_speed_t)
  calc plan start info and stitch trajectory1/2(plan_start_y) -> [plan_start_y_gcs]
  [obs_st_s_out_set] -> MATLAB Function5/6(obs_s_out_set)
  path and speed merge1/6(trajectory_accel) -> [trajectory_accel]
  generate convex space1/4(s_dot_ub) -> [s_dot_ub]
  Cartesian2Frenet3/1(Cartesian2FrenetOut) -> Bus Selector7/1
  [path_index2s] -> Cartesian2Frenet3/14(index2s)
  Frenet2Cartesian task/3(heading_set) -> [trajectory_heading_init]
  [obs_st_s_in_set] -> MATLAB Function5/5(obs_s_in_set)
  Constant56/1 -> path decision task1/13(dp_col)
  generate convex space1/2(s_ub) -> [s_ub]
  Constant50/1 -> generate convex space1/9(max_lateral_accel)
  path and speed merge1/3(trajectory_heading) -> [trajectory_heading]
  [obs_st_s_in_set] -> generate convex space1/4(obs_st_s_in_set)
  [host_ay_vcs] -> calc plan start info and stitch trajectory1/15(host_ay)
  [obs_st_t_out_set] -> generate convex space1/7(obs_st_t_out_set)
  [obs_st_s_in_set] -> speed decision with dynamic planning(dp)1/1(obs_st_s_in_set)
  Constant49/1 -> speed decision with dynamic planning(dp)1/8(w_cost_obs)
  [trajectory_kappa] -> stitch trajectory1/4(trajectory_kappa)
  [trajectory_y] -> stitch trajectory1/2(trajectory_y)
  [obs_st_t_out_set] -> speed decision with dynamic planning(dp)1/4(obs_st_t_out_set)
  [dynamic_obs_l_set] -> generate st graph1/4(dynamic_obs_l_set)
  [dp_speed_t] -> generate convex space1/2(dp_speed_t)
  [l_max] -> plot/6(l_max)
  calc plan start info and stitch trajectory1/5(plan_start_vx) -> [plan_start_vx_gcs]
  [qp_path_l_final] -> Frenet2Cartesian task/2(l_set)
  [s_lb] -> spee planning with quadratic programming (qp)/5(s_lb)
  Constant54/1 -> path decision task1/11(dp_cost_ref)
  Frenet2Cartesian task/2(y_set) -> [trajectory_y_init]
  generate st graph1/2(obs_st_s_out_set) -> [obs_st_s_out_set]
  [dynamic_obs_l_dot_set] -> generate st graph1/6(dynamic_obs_l_dot_set)
  MATLAB Function3/5(proj_kappa_set) -> Cartesian2Frenet3/13(proj_kappa_set)
  [dynamic_obs_s_set] -> generate st graph1/3(dynamic_obs_s_set)
  calc plan start info and stitch trajectory1/15(stitch_accel) -> [stitch_accel_gcs]
  [plan_start_ay_gcs] -> Cartesian2Frenet2/6(ay_set)
  generate st graph1/3(obs_st_t_in_set) -> [obs_st_t_in_set]
  [pre_trajectory_kappa_gcs] -> calc plan start info and stitch trajectory1/4(pre_trajectory_kappa)
  stitch trajectory1/7(trajectory_time_final) -> [trajectory_time_final]
  [relative_time] -> Delay3/1
  Constant32/1 -> path planning task1/20(delta_dl_max)
  Delay3/1 -> generate st graph1/2(pre_trajectory_t)
  obs1/2(static_obs_l_set) -> [static_obs_l_set]
  [plan_start_y_gcs] -> MATLAB Function4/2(y_set)
  [plan_start_l] -> path decision task1/4(plan_start_l)
  [trajectory_heading_init] -> MATLAB Function3/5(frenet_path_heading)
  [index2s] -> Frenet2Cartesian task/9(index2s)
  [trajectory_y_init] -> Cartesian2Frenet3/8(frenet_path_y)
  [pre_trajectory_y_gcs] -> calc plan start info and stitch trajectory1/2(pre_trajectory_y)
  [trajectory_x_init] -> Cartesian2Frenet3/7(frenet_path_x)
  stitch trajectory1/5(trajectory_speed_final) -> [trajectory_speed_final]
  [trajectory_x] -> stitch trajectory1/1(trajectory_x)
  path planning task1/3(qp_path_dl_final) -> [qp_path_dl_final]
  [obs_st_t_in_set] -> MATLAB Function5/7(obs_t_in_set)
  calc plan start info and stitch trajectory1/14(stitch_speed) -> [stitch_speed_gcs]
  Bus Selector7/2 -> [dynamic_obs_l_set]  "<l_set>"
  [trajectory_kappa_init] -> path and speed merge1/10(trajectory_kappa_init)
  [plan_start_vy_gcs] -> calc speed planning start condition1/2(plan_start_vy)
  [plan_start_vy_gcs] -> Cartesian2Frenet2/4(vy_set)
  MATLAB Function3/2(proj_x_set) -> Cartesian2Frenet3/10(proj_x_set)
  MATLAB Function3/4(proj_heading_set) -> Cartesian2Frenet3/12(proj_heading_set)
  [host_x] -> obs1/1(host_x)
  [pre_trajectory_accel_gcs] -> calc plan start info and stitch trajectory1/6(pre_trajectory_accel)
  MATLAB Function3/1(match_point_index_set) -> Cartesian2Frenet3/9(proj_match_point_index_set)
  Bus Selector7/4 -> [dynamic_obs_l_dot_set]  "<l_dot_set>"
  Ground3/1 -> Cartesian2Frenet3/6(ay_set)
  [stitch_time] -> stitch trajectory1/14(stitch_time)
  Ground2/1 -> Cartesian2Frenet3/5(ax_set)
  [dynamic_obs_x_set] -> Cartesian2Frenet3/1(x_set)
  [relative_time] -> path and speed merge1/4(relative_time)
  [l_min] -> plot/5(l_min)
  [s] -> Delay2/1
  [dynamic_obs_y_set] -> Cartesian2Frenet3/2(y_set)
  [obs_st_t_out_set] -> MATLAB Function5/8(obs_t_out_set)
  Selector17/1 -> [plan_start_dl]
  Constant41/1 -> path planning task1/16(qp_cost_end_ddl)
  obs1/4(dynamic_obs_y_set) -> [dynamic_obs_y_set]
  [qp_path_s_final] -> plot/3(qp_s)
  [plan_start_proj_y] -> Cartesian2Frenet2/11(proj_y_set)
  [obs_st_s_out_set] -> speed decision with dynamic planning(dp)1/2(obs_st_s_out_set)
  [qp_path_ddl_final] -> Frenet2Cartesian task/4(ddl_set)
  generate st graph1/4(obs_st_t_out_set) -> [obs_st_t_out_set]
  Constant55/1 -> path decision task1/12(dp_row)
  Constant42/1 -> path decision task1/9(dp_cost_ddl)
  calc plan start info and stitch trajectory1/11(stitch_y) -> [stitch_y_gcs]
  Constant33/1 -> path planning task1/21(delta_ddl_max)
  [dynamic_obs_y_set] -> MATLAB Function3/2(y_set)
  calc plan start info and stitch trajectory1/3(plan_start_heading) -> [plan_start_heading_gcs]
  [static_obs_l_set] -> path planning task1/4(static_obs_l_set)
  Constant31/1 -> path decision task1/8(dp_cost_dl)
  speed decision with dynamic planning(dp)1/1(dp_speed_s) -> [dp_speed_s]
  [plan_start_dl] -> path planning task1/7(plan_start_dl)
  calc speed planning start condition1/1(plan_start_s_dot) -> [plan_start_s_dot]
  calc plan start info and stitch trajectory1/10(stitch_x) -> [stitch_x_gcs]
  generate convex space1/1(s_lb) -> [s_lb]
  calc plan start info and stitch trajectory1/8(plan_start_ay) -> [plan_start_ay_gcs]
  [dynamic_obs_vy_set] -> Cartesian2Frenet3/4(vy_set)
  [s] -> path and speed merge1/1(s)
  [trajectory_y_init] -> MATLAB Function3/4(frenet_path_y)
  [qp_s_init] -> increase st point count1/1(s_init)
  path decision task1/4(dp_path_ddl_final) -> [dp_path_ddl_final]
  generate st graph1/1(obs_st_s_in_set) -> [obs_st_s_in_set]
  [stitch_heading_gcs] -> stitch trajectory1/10(stitch_heading)
  [plan_start_ax_gcs] -> calc speed planning start condition1/3(plan_start_ax)
  [dp_speed_s] -> MATLAB Function5/1(dp_speed_s)
  path planning task1/4(qp_path_ddl_final) -> [qp_path_ddl_final]
  [plan_start_ax_gcs] -> Cartesian2Frenet2/5(ax_set)
  [host_heading_xy] -> calc plan start info and stitch trajectory1/11(host_heading_xy)
  [trajectory_kappa_init] -> generate convex space1/8(trajectory_kappa_init)
  [trajectory_x_init] -> path and speed merge1/7(trajectory_x_init)
  [obs_st_t_in_set] -> generate convex space1/6(obs_st_t_in_set)
  obs1/3(dynamic_obs_x_set) -> [dynamic_obs_x_set]
  [relative_time_init] -> increase st point count1/4(relative_time_init)
  [stitch_speed_gcs] -> stitch trajectory1/12(stitch_speed)
  [plan_start_s_dot] -> speed decision with dynamic planning(dp)1/9(plan_start_s_dot)
  [reference_speed] -> speed decision with dynamic planning(dp)1/5(reference_speed_unlimit)
  [plan_start_s] -> path planning task1/5(plan_start_s)
  Bus Selector7/3 -> [dynamic_obs_s_dot_set]  "<s_dot_set>"
  [referenceline_x] -> genrate index to s/1(path_x)
  [qp_s_dot2_init] -> increase st point count1/3(s_dot2_init)
  [s_dot2] -> path and speed merge1/3(s_dot2)
  path and speed merge1/4(trajectory_kappa) -> [trajectory_kappa]
  [index2s] -> obs1/12(index2s)
  Constant46/1 -> [reference_speed]
  increase st point count1/3(s_dot2) -> [s_dot2]
  MATLAB Function4/1(match_point_index_set) -> Selector10/1
  [qp_path_s_final] -> Frenet2Cartesian task/1(s_set)
  [trajectory_kappa_init] -> MATLAB Function3/6(frenet_path_kappa)
  [dp_speed_t] -> MATLAB Function5/2(dp_speed_t)
  path planning task1/2(qp_path_l_final) -> [qp_path_l_final]
  [plan_start_vx_gcs] -> calc speed planning start condition1/1(plan_start_vx)
  [dp_speed_s] -> generate convex space1/1(dp_speed_s)
  [index2s] -> Cartesian2Frenet2/14(index2s)
  [host_x] -> calc plan start info and stitch trajectory1/9(host_x)
  Bus Selector7/1 -> [dynamic_obs_s_set]  "<s_set>"
  [referenceline_heading] -> MATLAB Function4/5(frenet_path_heading)
  [qp_path_dl_final] -> Frenet2Cartesian task/3(dl_set)
  Delay2/1 -> generate st graph1/1(pre_trajectory_s)
  [pre_trajectory_time] -> calc plan start info and stitch trajectory1/7(pre_trajectory_time)
  [s_dot] -> path and speed merge1/2(s_dot)
  [path_index2s] -> generate convex space1/3(path_index2s)
  Constant47/1 -> speed decision with dynamic planning(dp)1/6(w_cost_ref_speed)
  Constant43/1 -> path planning task1/17(host_d1)
  [relative_time_init] -> MATLAB Function5/4(qp_speed_t)
  MATLAB Function4/2(proj_x_set) -> Selector11/1
  [dynamic_obs_x_set] -> MATLAB Function3/1(x_set)
  Bus Selector6/3 -> Selector17/1  "<dl_set>"
  [s_ub] -> spee planning with quadratic programming (qp)/6(s_ub)
  path decision task1/3(dp_path_dl_final) -> [dp_path_dl_final]
  spee planning with quadratic programming (qp)/2(qp_s_dot_init) -> [qp_s_dot_init]
  [trajectory_x_init] -> MATLAB Function3/3(frenet_path_x)
  [trajectory_heading] -> stitch trajectory1/3(trajectory_heading)
  genrate index to s/1(index2s) -> [index2s]
  increase st point count1/2(s_dot) -> [s_dot]
  [plan_start_heading_gcs] -> calc speed planning start condition1/5(plan_start_heading)
  [qp_s_init] -> MATLAB Function5/3(qp_speed_s)
  [static_obs_s_set] -> path planning task1/3(static_obs_s_set)
  [dynamic_obs_vx_set] -> Cartesian2Frenet3/3(vx_set)
  [plan_start_l] -> path planning task1/6(plan_start_l)
  [trajectory_heading_init] -> path and speed merge1/9(trajectory_heading_init)
  Constant59/1 -> spee planning with quadratic programming (qp)/9(w_cost_s_dot2)
